simulink library "Library_2"  (R2024a)
settings: Solver=VariableStepAuto  StartTime=0.0  StopTime=10.0  RelTol=1e-3
undefined symbols (not defined in the file): a, am, b, bm, gamma
settings Model: Creator=marmr  LastModifiedBy=marmr

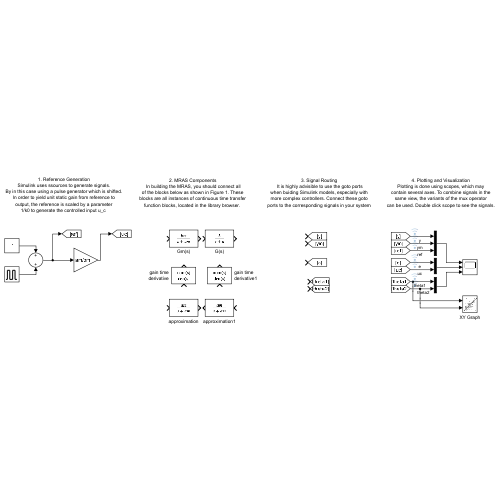
[thumbnail: Simulink's stored preview of the top-level diagram]
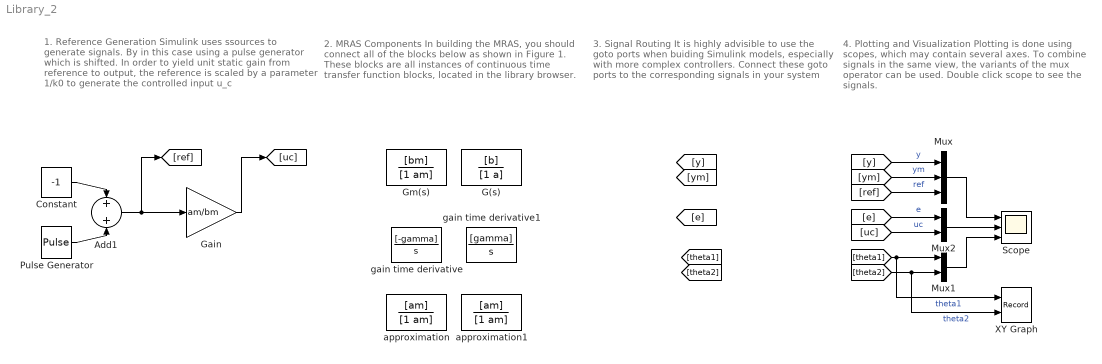
== system Library_2 ==
  note: 1. Reference Generation
      | Simulink uses ssources to generate signals.
      | By in this case using a pulse generator which is shifted.
      | In order to yield unit static gain from reference to
      | output, the reference is scaled by a parameter
      | 1/k0 to generate the controlled input u_c
  note: 4. Plotting and Visualization
      | Plotting is done using scopes, which may
      | contain several axes. To combine signals in the
      | same view, the variants of the mux operator
      | can be used. Double click scope to see the signals.
  note: 2. MRAS Components
      |  In building the MRAS, you should connect all
      | of the blocks below as shown in Figure 1. These
      | blocks are all instances of continuous time transfer
      | function blocks, located in the library browser.
  note: 3. Signal Routing
      |  It is highly advisible to use the goto ports
      | when buiding Simulink models, especially with
      | more complex controllers. Connect these goto
      | ports to the corresponding signals in your system
  Add1 : Sum
  Constant : Constant  Value=-1  SampleTime=0.1
  G(s) : TransferFcn  Numerator=[b]  Denominator=[1 a]
  Gain : Gain  Gain=am/bm
  Gm(s) : TransferFcn  Numerator=[bm]  Denominator=[1 am]
  Mux : Mux  Inputs=3
  Mux1 : Mux  Inputs=2
  Mux2 : Mux  Inputs=2
  Pulse Generator : DiscretePulseGenerator  PulseType=Time based  Amplitude=2  Period=10  PulseWidth=50
  Scope : Scope  NumInputPorts=3
  XY Graph : Record  FileSettingsInternal="{\"entries\":[{\"content\":{\"excelSettings\":{\"content\":{},\"type\":\"Streamout.ExcelSettings\"}},\"type\":\"Streamout.FileSettingStorage\",\"uuid\":\"\"}],\"packageUris\":[\"http:\\/\\/schema.mathworks.com\\/mf0\\/streamout_blocks\\/R2020a\"],\"version\":\"1.0\"}"  Layout=[1 1]  SignalsInternal="{\"entries\":[{\"content\":{\"signals\":[{\"content\":{\"blockPath\":[],\"dimensions\":[1],\"domain\":\"\",\"lineColor\":\"#a2142f\",\"plots\":[ 1 ],\"port\":1,\"signalID\":1,\"signalName\":\"     \"},\"type\":\"RecordBlkView.Signal\",\"uuid\":\"\"},{\"content\":{\"blockPath\":[],\"dimensions\":[1],\"domain\":\"\",\"lineColor\":\"#139fff\",\"plots\":[ 1 ],\"port\":2,\"signalID\":2,\"signalName\":\"              \"},\"type\":\"RecordBlkView.Signal\",\"uuid\":\"\"}]},\"type\":\"RecordBlkView.InputSignals\",\"uuid\":\"\"}],\"packageUris\":[\"http:\\/\\/schema.mathworks.com\\/mf0\\/streamout_blocks\\/R2020a\"],\"version\":\"1.0\"}"  VisualizationBindings="{\"xyplotplugin\":{\"info\":[{\"series\":[{\"bindingParametersList\":[{\"parameter\":\"X-Axis\",\"signalID\":1,\"signalName\":\"     \"},{\"parameter\":\"Y-Axis\",\"signalID\":2,\"signalName\":\"              \"}],\"seriesID\":0}],\"subplotID\":1}]}}"  CompatibilityTag=XY  st=-1
  approximation : TransferFcn  Numerator=[am]  Denominator=[1 am]
  approximation1 : TransferFcn  Numerator=[am]  Denominator=[1 am]
  gain time derivative : TransferFcn  Numerator=[-gamma]  Denominator=[1 0]
  gain time derivative1 : TransferFcn  Numerator=[gamma]  Denominator=[1 0]
  wires:
  Mux/1 -> Scope/1
  Gain/1 -> [uc]
  [theta1] -> Mux1/1, XY Graph/1  "theta1"
  [ym] -> Mux/2  "ym"
  [e] -> Mux2/1  "e"
  [ref] -> Mux/3  "ref"
  Add1/1 -> Gain/1, [ref]
  Mux2/1 -> Scope/2
  Mux1/1 -> Scope/3
  [theta2] -> Mux1/2, XY Graph/2  "theta2"
  Pulse Generator/1 -> Add1/2
  Constant/1 -> Add1/1
  [y] -> Mux/1  "y"
  [uc] -> Mux2/2  "uc"
